simulink model "Jxerr"  (R2019b)
settings: Solver=VariableStepAuto  StartTime=0.0  StopTime=7  RelTol=1e-3
values from neighbouring files (symbols this model uses):
  des_E = [20*scale; 140*scale; 290*scale]    [init.m]
  par = [a1, a2, a3, d1]    [init.m]
  q0 = [deg2rad(0); deg2rad(90); deg2rad(-90)]    [init.m]
  Ts = 0.1    [init.m]
undefined symbols (not defined in the file or in its folder): DiscIntNeverNeededParam
settings Model: Creator=Matteo  LastModifiedBy=matteo
settings SolverCC: AlgebraicLoopSolver=LineSearch

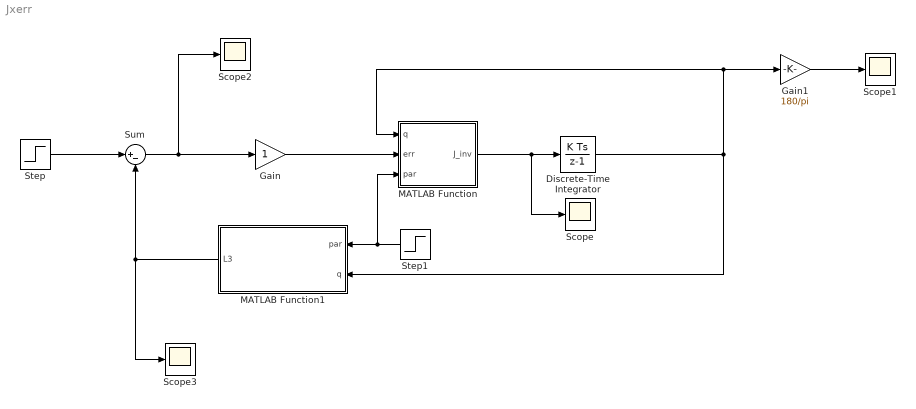
== system Jxerr ==
  Discrete-Time Integrator : DiscreteIntegrator  InitialCondition=q0  SampleTime=Ts  ICPrevOutput=DiscIntNeverNeededParam  ICPrevScaledInput=DiscIntNeverNeededParam
  Gain : Gain
  Gain1 : Gain  Gain=180/pi
  MATLAB Function : MATLAB Function  TreatAsAtomicUnit=on
  MATLAB Function1 : MATLAB Function  TreatAsAtomicUnit=on
  Scope{,1..3} (4 alike) : Scope
  Step : Step  Time=0  After=des_E  SampleTime=0
  Step1 : Step  Time=0  After=par  SampleTime=0
  Sum : Sum  Inputs=|+-
  wires:
  Step/1 -> Sum/1
  Sum/1 -> Gain/1, Scope2/1
  MATLAB Function/1(J_inv) -> Discrete-Time Integrator/1, Scope/1
  MATLAB Function1/1(L3) -> Scope3/1, Sum/2
  Discrete-Time Integrator/1 -> MATLAB Function1/2(q), MATLAB Function/1(q), Gain1/1
  Gain1/1 -> Scope1/1
  Step1/1 -> MATLAB Function1/1(par), MATLAB Function/3(par)
  Gain/1 -> MATLAB Function/2(err)

== matlab function Jxerr/MATLAB Function1 ==
  data: par input; q input; L3 output
function L3 = direct_kynematics(par, q)
    th1 = q(1); th2 = q(2); th3 = q(3); a1 = par(1); a2 = par(2); a3 = par(3); d1 = par(4);
    L1 = [-a1*sin(th1); a1*cos(th1); d1];
    L2 = L1 + [-a2*cos(th2)*sin(th1); a2*cos(th2)*cos(th1); a2*sin(th2)];
    L3 = L2 + [-a3*cos(th2+th3)*sin(th1); a3*cos(th2+th3)*cos(th1); a3*sin(th2+th3)];
    
end

== matlab function Jxerr/MATLAB Function ==
  data: q input; J_inv output; err input; par input
function J_inv = jacobian(q, err, par)
scale = 1;
des_E = [20*scale; 140*scale; 290*scale]; % POSIZIONE DESIDERATA DELL'END-EFFECTOR
start_E = [0*scale; 160*scale; 290*scale];

    S = [des_E(1)-start_E(1);
         des_E(2)-start_E(2);
         des_E(3)-start_E(3)];
    vel = 25;
    th1 = q(1); th2 = q(2); th3 = q(3); a1 = par(1); a2 = par(2); a3 = par(3);
    Ja = [-cos(th1)*(a1+a2*cos(th2)+a3*cos(th2+th3)), sin(th1)*(a2*sin(th2)+a3*sin(th2+th3)),sin(th1)*a3*sin(th2+th3);
         -sin(th1)*(a1+a2*cos(th2)+a3*cos(th2+th3)), -cos(th1)*(a2*sin(th2)+a3*sin(th2+th3)),-cos(th1)*a3*sin(th2+th3);
         0                                          , a2*cos(th2)+a3*cos(th2+th3)            , a3*cos(th2+th3)];
%     J_inv = Ja\err;
    J_inv = Ja\S*(vel/norm(S));
end
